simulink model "Smart_City_QCar1_self_driving_stack"  (R2024b)
settings: Solver=ode1  StartTime=0.0  StopTime=inf  FixedStep=Controller_Sample_Time  RelTol=1e-3  EnableMultiTasking=on
values from neighbouring files (symbols this model uses):
  angles_qcar1 = angles_new_qcar1(2: length (angles_new_qcar1), width (angles_new_qcar1)-5)    [Setup_QCar1and2_params.m]
  Audio_Sample_Time = 0.3    [Setup_QCar1and2_params.m]
  cal_pos = [0, 0, 0]    [Setup_QCar1and2_params.m]
  cameraStepSize = 3e-2    (= 0.03)    [Setup_QCar1and2_params.m]
  Cobra_Start = [0 0 0 0 0 0 0 0 0 0 0 0 ... (192000 elements, 192000x1)]    [QCar_Sounds.mat]
  Controller_Sample_Time = CSI_Sample_Time/10    (= 0.00166666666667)    [Setup_QCar1and2_params.m]
  CSI_Sample_Time = 1/60    (= 0.0166666666667)    [Setup_QCar1and2_params.m]
  GyroKF_P0 = eye(2)    [Setup_QCar1and2_params.m]
  GyroKF_Q = diag([0.01, 0.001])    [Setup_QCar1and2_params.m]
  GyroKF_R = 0.01    [Setup_QCar1and2_params.m]
  GyroKF_X0 = [0;0]    [Setup_QCar1and2_params.m]
  honk = [0.01708984375 0.0179443359375 0.018798828125 0.019775390625 0.0209655761719 0.0218505859375 0.0221557617188 0.0223693847656 0.022705078125 0.023681640625 0.0252075195312 0.0257263183594 ... (43568 elements, 21784x2)]    [QCar_Sounds.mat]
  ImageDisplay_Sample_Time = CSI_Sample_Time*6    (= 0.1)    [Setup_QCar1and2_params.m]
  Initialization_Time = 5    [Setup_QCar1and2_params.m]
  LiDAR_Sample_Time = CSI_Sample_Time*3    (= 0.05)    [Setup_QCar1and2_params.m]
  map_mask = [1 1 1 0 0 1 0]    [Setup_QCar1and2_params.m]
  NN_Sample_Time = RealSense_Sample_Time*1    (= 0.0333333333333)    [Setup_QCar1and2_params.m]
  path_x = [0.826 0.836 0.846 0.856 0.866 0.876 0.886 0.896 0.906 0.916 0.926 0.936 ... (740 elements, 740x1)]    [SDCS_Paths_7.mat]
  path_x2 = [-0.614 -0.604 -0.594 -0.584 -0.574 -0.564 -0.554 -0.544 -0.534 -0.524 -0.514 -0.504 ... (1090 elements, 1090x1)]    [SDCS_Paths_7.mat]
  path_x3 = [-0.614 -0.603821428571 -0.593642857143 -0.583464285714 -0.573285714286 -0.563107142857 -0.552928571429 -0.54275 -0.532571428571 -0.522392857143 -0.512214285714 -0.502035714286 ... (714 elements, 714x1)]    [SDCS_Paths_7.mat]
  path_x4 = [-0.614 -0.604 -0.594 -0.584 -0.574 -0.564 -0.554 -0.544 -0.534 -0.524 -0.514 -0.504 ... (1761 elements, 1761x1)]    [SDCS_Paths_7.mat]
  path_x5 = [1.436 1.42588571429 1.41577142857 1.40565714286 1.39554285714 1.38542857143 1.37531428571 1.3652 1.35508571429 1.34497142857 1.33485714286 1.32474285714 ... (574 elements, 574x1)]    [SDCS_Paths_7.mat]
  path_x6 = [1.436 1.42588571429 1.41577142857 1.40565714286 1.39554285714 1.38542857143 1.37531428571 1.3652 1.35508571429 1.34497142857 1.33485714286 1.32474285714 ... (1288 elements, 1288x1)]    [SDCS_Paths_7.mat]
  path_x7 = [-1.5778487585 -1.56959877056 -1.56127865467 -1.55288878259 -1.54442952915 -1.53590127231 -1.52730439309 -1.51863927561 -1.50990630701 -1.50110587746 -1.49223838016 -1.4833042113 ... (2260 elements, 2260x1)]    [SDCS_Paths_7.mat]
  path_y = [-1.0887 -1.0887 -1.0887 -1.0887 -1.0887 -1.0887 -1.0887 -1.0887 -1.0887 -1.0887 -1.0887 -1.0887 ... (740 elements, 740x1)]    [SDCS_Paths_7.mat]
  path_y2 = [-1.0887 -1.0887 -1.0887 -1.0887 -1.0887 -1.0887 -1.0887 -1.0887 -1.0887 -1.0887 -1.0887 -1.0887 ... (1090 elements, 1090x1)]    [SDCS_Paths_7.mat]
  path_y3 = [-1.0887 -1.0887 -1.0887 -1.0887 -1.0887 -1.0887 -1.0887 -1.0887 -1.0887 -1.0887 -1.0887 -1.0887 ... (714 elements, 714x1)]    [SDCS_Paths_7.mat]
  path_y4 = [-1.0887 -1.0887 -1.0887 -1.0887 -1.0887 -1.0887 -1.0887 -1.0887 -1.0887 -1.0887 -1.0887 -1.0887 ... (1761 elements, 1761x1)]    [SDCS_Paths_7.mat]
  path_y5 = [-0.8157 -0.8157 -0.8157 -0.8157 -0.8157 -0.8157 -0.8157 -0.8157 -0.8157 -0.8157 -0.8157 -0.8157 ... (574 elements, 574x1)]    [SDCS_Paths_7.mat]
  path_y6 = [-0.8157 -0.8157 -0.8157 -0.8157 -0.8157 -0.8157 -0.8157 -0.8157 -0.8157 -0.8157 -0.8157 -0.8157 ... (1288 elements, 1288x1)]    [SDCS_Paths_7.mat]
  path_y7 = [-0.614490295955 -0.61974988896 -0.624981792226 -0.630185771997 -0.635361595765 -0.640509032279 -0.645627851559 -0.6507178249 -0.655778724888 -0.660810325409 -0.665812401655 -0.670784730139 ... (2260 elements, 2260x1)]    [SDCS_Paths_7.mat]
  put_me_down = [0 0 0 0 0 0 0 0 0 0 0 0 ... (335870 elements, 167935x2)]    [QCar_Sounds.mat]
  qcar1_lidar_to_map_rotation = pi/2    (= 1.57079632679)    [Setup_QCar1and2_params.m]
  QCarEKF_L = 0.24    [Setup_QCar1and2_params.m]
  QCarEKF_P0 = eye(3)    [Setup_QCar1and2_params.m]
  QCarEKF_Q = diag([0.00001, 0.00001, 0.00001])    [Setup_QCar1and2_params.m]
  QCarEKF_R_combined = diag([0.1, 0.1, 0.01])    [Setup_QCar1and2_params.m]
  QCarEKF_R_heading = diag(0.1)    [Setup_QCar1and2_params.m]
  QcarKF_X0 = [0; 0; 0]    [Setup_QCar1and2_params.m]
  range_qcar1 = distance_new_qcar1(2: length (distance_new_qcar1), width (distance_new_qcar1)-5)    [Setup_QCar1and2_params.m]
  RealSense_Sample_Time = CSI_Sample_Time*2    (= 0.0333333333333)    [Setup_QCar1and2_params.m]
undefined symbols (not defined in the file or in its folder): DiscIntNeverNeededParam, gcbh, HIL, Joystick_Sample_Time, JPEG, Point, qc_get_step_size, video_display_show
libraries: quarc_library x63, simulink_extras x12, simulink x8
(part 2 of 5)

== system Smart_City_QCar1_self_driving_stack/QCar/QCar Control ==
  "Command (m/s, rad)" : Inport
  Model Heading (rad) : Inport  Port=2
  Hazard : Inport  Port=3
  Cos ^ : Inport  Port=4
  Car on : Inport  Port=5
  acceleration : Inport  Port=6
  Volume : Inport  Port=7
  Honk : Inport  Port=8
  Command : Saturate  UpperLimit=[3 .6]  LowerLimit=-[3 .6]
  Constant5 : Constant  Value=-inf
  Constant6 : Constant
  Data Type Conversion : DataTypeConversion  SaturateOnIntegerOverflow=off  RndMeth=Floor
  Demux : Demux  Outputs=2
  Demux1 : Demux  Outputs=2
  Display : Display
      settings: Decimation=100
  Display1 : Display
      settings: Decimation=100
  Memory : Memory
  Mux : Mux  Inputs=2
  Mux1 : Mux  Inputs=2
  Product : Product
  QCar I/O : Subsystem
  Rate Limiter Dynamic : simulink/Discontinuities/Rate Limiter Dynamic
  bicycleModel : Subsystem
  powerConsumptionMonitor : Subsystem
  speedController : Subsystem
  turnSpeedHandling : Subsystem
  Car Speed (m/s) : Outport
  "Pose_dot (m/s, m/s, rad/s)" : Outport  Port=2
  Battery (V) : Outport  Port=3
  Odometer (m) : Outport  Port=4
  Actual Steering : Outport  Port=5
  Current (A) : Outport  Port=6
  Commanded Speed : Outport  Port=7
  Gyro (rad/s) : Outport  Port=8
  wires:
  QCar I/O/2(batteryVoltage (V) [1]) -> Battery (V)/1, powerConsumptionMonitor/2(batteryVoltage (V) [1])
  powerConsumptionMonitor/1(motorPowerConsumption (W) [1]) -> Display/1
  QCar I/O/1(motorCurrent (A) [1]) -> Current (A)/1, powerConsumptionMonitor/1(motorCurrent (A) [1])
  Model Heading (rad)/1 -> bicycleModel/1(heading (rad))
  powerConsumptionMonitor/2(batteryLevel (%) [1]) -> Display1/1
  QCar I/O/4(gyroscopicRates (rad/s)) -> Gyro (rad/s)/1, bicycleModel/4(gyroscope (rad/s))
  bicycleModel/1("poseRate (m/s, m/s, rad/s)") -> "Pose_dot (m/s, m/s, rad/s)"/1
  Product/1 -> QCar I/O/1("motorCmd (%, rad) [2]"), bicycleModel/2("motorCommands (%, rad)"), Demux/1
  Car on/1 -> QCar I/O/2(Arm), speedController/1(arm (0,1)), Mux/1
  QCar I/O/5(Odometer) -> Odometer (m)/1
  [Speed] -> speedController/3(measuredSpeed (m/s))
  Demux/2 -> Actual Steering/1
  Hazard/1 -> Data Type Conversion/1
  Cos ^/1 -> turnSpeedHandling/2(Cos ^)
  Data Type Conversion/1 -> QCar I/O/3(Hazard)
  speedController/1(throttleCmd (%)) -> Product/2
  Mux/1 -> Product/1
  Constant6/1 -> Mux/2
  Volume/1 -> QCar I/O/4(Volume)
  QCar I/O/3(Speed (m/s)) -> [Speed], bicycleModel/3(carSpeed (m/s)), Car Speed (m/s)/1  "v"
  "Command (m/s, rad)"/1 -> Command/1
  Demux1/1 -> Rate Limiter Dynamic/2
  Rate Limiter Dynamic/1 -> Memory/1, Mux1/1
  Constant5/1 -> Rate Limiter Dynamic/3
  acceleration/1 -> Rate Limiter Dynamic/1
  Demux1/2 -> Mux1/2
  turnSpeedHandling/1(Commands) -> Demux1/1
  Mux1/1 -> speedController/2(desiredSpeed (m/s))
  Command/1 -> turnSpeedHandling/1(Commands in)
  Honk/1 -> QCar I/O/5(Honk)
  Memory/1 -> Commanded Speed/1

== system Smart_City_QCar1_self_driving_stack/QCar/QCar State Estimation ==
  v : Inport
  delta : Inport  Port=2
  x_gps : Inport  Port=3
  y_gps : Inport  Port=4
  th_gps : Inport  Port=5
  thd_gyro : Inport  Port=6
  newGPSData : Inport  Port=7
  Gyro Kalman Filter : MATLAB Function  TreatAsAtomicUnit=on
  QCar EKF : MATLAB Function  TreatAsAtomicUnit=on
  Xhat : Outport
  gyro_bias : Outport  Port=2
  wires:
  x_gps/1 -> QCar EKF/3(x_gps)
  y_gps/1 -> QCar EKF/4(y_gps)
  Gyro Kalman Filter/1(th_hat) -> QCar EKF/5(th_hat)
  newGPSData/1 -> QCar EKF/6(newGPSData), Gyro Kalman Filter/3(newGPSData)
  delta/1 -> QCar EKF/2(delta)
  thd_gyro/1 -> Gyro Kalman Filter/1(thd_gyro)
  v/1 -> QCar EKF/1(v)
  QCar EKF/1(Xhat) -> Xhat/1
  th_gps/1 -> Gyro Kalman Filter/2(th_gps)
  Gyro Kalman Filter/2(gyro_bias) -> gyro_bias/1

== system Smart_City_QCar1_self_driving_stack/QCar/Sensor Fusion - Complementary Filter ==
  note: One idead is to have the integrator reset if rate is high...
  note: stable gains Kp = 0.4*.4
  car speed : Inport
  rate : Inport  Port=2
  correction : Inport  Port=3
  Constant : Constant
  Constant1 : Constant  Value=5
  Constant2 : Constant  Value=.1
  Correction_Weight : Scope
  Display : Display
  Gain : Gain  Gain=[100 100 1]
  Integrator : Integrator  WrappedStateUpperValue=[20 20 pi]  WrappedStateLowerValue=-[20 20 pi]
  Integrator1 : Integrator  ExternalReset=level  LimitOutput=on  UpperSaturationLimit=.05*[1 1 1]*1  LowerSaturationLimit=-.05*[1 1 1]*1
  MATLAB Function : MATLAB Function  TreatAsAtomicUnit=on
  Manual Switch : ManualSwitch  CurrentSetting=0
  Product : Product
  Scope : Scope  NumInputPorts=2
  Subtract : Sum  Inputs=+-
  Subtract1 : Sum  Inputs=+-
  Subtract2 : Sum
  ki : Gain  Gain=[4 4 4]*1
  kp : Gain  Gain=[1 1 1]*.400*1
  estimate : Outport  VectorParamsAs1DForOutWhenUnconnected=off
  wires:
  Integrator/1 -> Subtract/1, estimate/1
  Subtract/1 -> ki/1, kp/1
  Integrator1/1 -> Scope/1, Subtract2/2
  kp/1 -> Scope/2, Subtract2/1
  Subtract1/1 -> Integrator/1
  ki/1 -> Integrator1/1
  correction/1 -> Subtract/2
  rate/1 -> Subtract1/1
  Manual Switch/1 -> Integrator1/2
  Constant/1 -> Manual Switch/1
  car speed/1 -> MATLAB Function/1(car_speed)
  MATLAB Function/1(correction_weight) -> Correction_Weight/1, Product/1, Display/1
  Subtract2/1 -> Gain/1
  Product/1 -> Subtract1/2
  Constant1/1 -> MATLAB Function/2(slope)
  Constant2/1 -> MATLAB Function/3(min_weight)
  Gain/1 -> Product/2

== system Smart_City_QCar1_self_driving_stack/QCar/Subsystem ==
  Angle : Inport
  Bias : Bias  Bias=pi  SaturateOnIntegerOverflow=off
  Bias1 : Bias  Bias=-pi  SaturateOnIntegerOverflow=off
  Constant1 : Constant  Value=2*pi
  Mod : Math  Operator=mod  SignedPower=on
  Mod_Angle : Outport
  wires:
  Mod/1 -> Bias1/1
  Constant1/1 -> Mod/2
  Bias/1 -> Mod/1
  Bias1/1 -> Mod_Angle/1
  Angle/1 -> Bias/1

== system Smart_City_QCar1_self_driving_stack/QCar/Subsystem1 ==
  Angle : Inport
  Bias : Bias  Bias=pi  SaturateOnIntegerOverflow=off
  Bias1 : Bias  Bias=-pi  SaturateOnIntegerOverflow=off
  Constant1 : Constant  Value=2*pi
  Mod : Math  Operator=mod  SignedPower=on
  Mod_Angle : Outport
  wires:
  Angle/1 -> Bias/1
  Bias1/1 -> Mod_Angle/1
  Bias/1 -> Mod/1
  Constant1/1 -> Mod/2
  Mod/1 -> Bias1/1

== system Smart_City_QCar1_self_driving_stack/Randomizer1/Subsystem1 ==
  Random Period : Inport
  Constant1 : Constant
  Less Than : RelationalOperator  Operator=<  OutDataTypeStr=boolean  RndMeth=Simplest  InputSameDT=off
  Mod : Math  Operator=mod
  Rate Transition : RateTransition  OutPortSampleTime=qc_get_step_size
  RisingEdge : Subsystem
  Time : quarc_library/Sources/Time/Time  time_source=Wall clock  sample_time=cameraStepSize*10
  RisingEdgeTrigger : Outport
  wires:
  Mod/1 -> Less Than/1
  Constant1/1 -> Less Than/2
  Rate Transition/1 -> Mod/1
  Less Than/1 -> RisingEdge/1(Input)
  Random Period/1 -> Mod/2
  Time/1 -> Rate Transition/1
  RisingEdge/1(RisingEdgeTrigger) -> RisingEdgeTrigger/1

== system Smart_City_QCar1_self_driving_stack/Randomizer1/select which which path set to use ==
  Trigger : TriggerPort  VariantControl=(inherit)
  Constant : Constant  Value=[1 1 0 1 0 0 1]
  Constant1 : Constant  Value=[0 0 1 0 1 1 0]
  Random Number : RandomNumber  Seed=7
  Switch : Switch  Criteria=u2 > Threshold  SaturateOnIntegerOverflow=off  InputSameDT=off
  map mask : Outport
  wires:
  Random Number/1 -> Switch/2
  Constant/1 -> Switch/1
  Constant1/1 -> Switch/3
  Switch/1 -> map mask/1

== system Smart_City_QCar1_self_driving_stack/Rate Timing Plots/monitorTiming ==
  note: Timing Performance
  note: moniorTiming Module:
      |
      | This subsystem outputs the sample time and computation time of the model.
      |
      | Outputs:
      | sampleTime (s) n/a : Sample time (unfiltered and filtered) in seconds.
      | computationTime (s) n/a : Computation time (unfiltered and filtered) in seconds.
      |
      | Usage:
      | Compare the Sample Time (s) output to a constant (qc_get_step_size) to monitor whether or not the desired sample time is being achieved. The Computation Time (s) values should be lower than the corresponding sample time value to ensure that the solver has enough time per time step.
  Computation Time : quarc_library/Sources/Time/Computation Time  sample_time=CSI_Sample_Time  use_model=on  use_cpu_time=off
  Constant : Constant  Value=CSI_Sample_Time  SampleTime=-1
  Mux : Mux  Inputs=3
  Sample Time : quarc_library/Sources/Time/Sample Time  Priority=-99  sample_time=CSI_Sample_Time
  Timing (s) : Outport  VectorParamsAs1DForOutWhenUnconnected=off
  wires:
  Computation Time/1 -> Mux/3
  Mux/1 -> Timing (s)/1
  Sample Time/1 -> Mux/1
  Constant/1 -> Mux/2

== system Smart_City_QCar1_self_driving_stack/Rate Timing Plots/monitorTiming1 ==
  note: moniorTiming Module:
      |
      | This subsystem outputs the sample time and computation time of the model.
      |
      | Outputs:
      | sampleTime (s) n/a : Sample time (unfiltered and filtered) in seconds.
      | computationTime (s) n/a : Computation time (unfiltered and filtered) in seconds.
      |
      | Usage:
      | Compare the Sample Time (s) output to a constant (qc_get_step_size) to monitor whether or not the desired sample time is being achieved. The Computation Time (s) values should be lower than the corresponding sample time value to ensure that the solver has enough time per time step.
  note: Timing Performance
  Computation Time : quarc_library/Sources/Time/Computation Time  sample_time=qc_get_step_size  use_model=on  use_cpu_time=off
  Constant : Constant  Value=qc_get_step_size  SampleTime=-1
  Mux : Mux  Inputs=3
  Sample Time : quarc_library/Sources/Time/Sample Time  Priority=-99  sample_time=qc_get_step_size
  Timing (s) : Outport  VectorParamsAs1DForOutWhenUnconnected=off
  wires:
  Constant/1 -> Mux/2
  Sample Time/1 -> Mux/1
  Mux/1 -> Timing (s)/1
  Computation Time/1 -> Mux/3

== system Smart_City_QCar1_self_driving_stack/Rate Timing Plots/monitorTiming2 ==
  note: moniorTiming Module:
      |
      | This subsystem outputs the sample time and computation time of the model.
      |
      | Outputs:
      | sampleTime (s) n/a : Sample time (unfiltered and filtered) in seconds.
      | computationTime (s) n/a : Computation time (unfiltered and filtered) in seconds.
      |
      | Usage:
      | Compare the Sample Time (s) output to a constant (qc_get_step_size) to monitor whether or not the desired sample time is being achieved. The Computation Time (s) values should be lower than the corresponding sample time value to ensure that the solver has enough time per time step.
  note: Timing Performance
  Computation Time : quarc_library/Sources/Time/Computation Time  sample_time=RealSense_Sample_Time  use_model=on  use_cpu_time=off
  Constant : Constant  Value=RealSense_Sample_Time  SampleTime=-1
  Mux : Mux  Inputs=3
  Sample Time : quarc_library/Sources/Time/Sample Time  Priority=-99  sample_time=RealSense_Sample_Time
  Timing (s) : Outport  VectorParamsAs1DForOutWhenUnconnected=off
  wires:
  Constant/1 -> Mux/2
  Sample Time/1 -> Mux/1
  Mux/1 -> Timing (s)/1
  Computation Time/1 -> Mux/3

== system Smart_City_QCar1_self_driving_stack/Rate Timing Plots/monitorTiming3 ==
  note: Timing Performance
  note: moniorTiming Module:
      |
      | This subsystem outputs the sample time and computation time of the model.
      |
      | Outputs:
      | sampleTime (s) n/a : Sample time (unfiltered and filtered) in seconds.
      | computationTime (s) n/a : Computation time (unfiltered and filtered) in seconds.
      |
      | Usage:
      | Compare the Sample Time (s) output to a constant (qc_get_step_size) to monitor whether or not the desired sample time is being achieved. The Computation Time (s) values should be lower than the corresponding sample time value to ensure that the solver has enough time per time step.
  Computation Time : quarc_library/Sources/Time/Computation Time  sample_time=ImageDisplay_Sample_Time  use_model=on  use_cpu_time=off
  Constant : Constant  Value=ImageDisplay_Sample_Time  SampleTime=-1
  Mux : Mux  Inputs=3
  Sample Time : quarc_library/Sources/Time/Sample Time  Priority=-99  sample_time=ImageDisplay_Sample_Time
  Timing (s) : Outport  VectorParamsAs1DForOutWhenUnconnected=off
  wires:
  Computation Time/1 -> Mux/3
  Mux/1 -> Timing (s)/1
  Sample Time/1 -> Mux/1
  Constant/1 -> Mux/2

== system Smart_City_QCar1_self_driving_stack/Rate Timing Plots/monitorTiming4 ==
  note: Timing Performance
  note: moniorTiming Module:
      |
      | This subsystem outputs the sample time and computation time of the model.
      |
      | Outputs:
      | sampleTime (s) n/a : Sample time (unfiltered and filtered) in seconds.
      | computationTime (s) n/a : Computation time (unfiltered and filtered) in seconds.
      |
      | Usage:
      | Compare the Sample Time (s) output to a constant (qc_get_step_size) to monitor whether or not the desired sample time is being achieved. The Computation Time (s) values should be lower than the corresponding sample time value to ensure that the solver has enough time per time step.
  Computation Time : quarc_library/Sources/Time/Computation Time  sample_time=Joystick_Sample_Time  use_model=on  use_cpu_time=off
  Constant : Constant  Value=Joystick_Sample_Time  SampleTime=-1
  Mux : Mux  Inputs=3
  Sample Time : quarc_library/Sources/Time/Sample Time  Priority=-99  sample_time=Joystick_Sample_Time
  Timing (s) : Outport  VectorParamsAs1DForOutWhenUnconnected=off
  wires:
  Computation Time/1 -> Mux/3
  Mux/1 -> Timing (s)/1
  Sample Time/1 -> Mux/1
  Constant/1 -> Mux/2

== system Smart_City_QCar1_self_driving_stack/Rate Timing Plots/monitorTiming5 ==
  note: moniorTiming Module:
      |
      | This subsystem outputs the sample time and computation time of the model.
      |
      | Outputs:
      | sampleTime (s) n/a : Sample time (unfiltered and filtered) in seconds.
      | computationTime (s) n/a : Computation time (unfiltered and filtered) in seconds.
      |
      | Usage:
      | Compare the Sample Time (s) output to a constant (qc_get_step_size) to monitor whether or not the desired sample time is being achieved. The Computation Time (s) values should be lower than the corresponding sample time value to ensure that the solver has enough time per time step.
  note: Timing Performance
  Computation Time : quarc_library/Sources/Time/Computation Time  sample_time=LiDAR_Sample_Time  use_model=on  use_cpu_time=off
  Constant : Constant  Value=LiDAR_Sample_Time  SampleTime=-1
  Mux : Mux  Inputs=3
  Sample Time : quarc_library/Sources/Time/Sample Time  Priority=-99  sample_time=LiDAR_Sample_Time
  Timing (s) : Outport  VectorParamsAs1DForOutWhenUnconnected=off
  wires:
  Constant/1 -> Mux/2
  Sample Time/1 -> Mux/1
  Mux/1 -> Timing (s)/1
  Computation Time/1 -> Mux/3

== system Smart_City_QCar1_self_driving_stack/Rate Timing Plots/monitorTiming6 ==
  note: Timing Performance
  note: moniorTiming Module:
      |
      | This subsystem outputs the sample time and computation time of the model.
      |
      | Outputs:
      | sampleTime (s) n/a : Sample time (unfiltered and filtered) in seconds.
      | computationTime (s) n/a : Computation time (unfiltered and filtered) in seconds.
      |
      | Usage:
      | Compare the Sample Time (s) output to a constant (qc_get_step_size) to monitor whether or not the desired sample time is being achieved. The Computation Time (s) values should be lower than the corresponding sample time value to ensure that the solver has enough time per time step.
  Computation Time : quarc_library/Sources/Time/Computation Time  sample_time=NN_Sample_Time  use_model=on  use_cpu_time=off
  Constant : Constant  Value=NN_Sample_Time  SampleTime=-1
  Mux : Mux  Inputs=3
  Sample Time : quarc_library/Sources/Time/Sample Time  Priority=-99  sample_time=NN_Sample_Time
  Timing (s) : Outport  VectorParamsAs1DForOutWhenUnconnected=off
  wires:
  Computation Time/1 -> Mux/3
  Mux/1 -> Timing (s)/1
  Sample Time/1 -> Mux/1
  Constant/1 -> Mux/2

== system Smart_City_QCar1_self_driving_stack/Rate Timing Plots/monitorTiming7 ==
  note: Timing Performance
  note: moniorTiming Module:
      |
      | This subsystem outputs the sample time and computation time of the model.
      |
      | Outputs:
      | sampleTime (s) n/a : Sample time (unfiltered and filtered) in seconds.
      | computationTime (s) n/a : Computation time (unfiltered and filtered) in seconds.
      |
      | Usage:
      | Compare the Sample Time (s) output to a constant (qc_get_step_size) to monitor whether or not the desired sample time is being achieved. The Computation Time (s) values should be lower than the corresponding sample time value to ensure that the solver has enough time per time step.
  Computation Time : quarc_library/Sources/Time/Computation Time  sample_time=1  use_model=on  use_cpu_time=off
  Constant : Constant  SampleTime=-1
  Mux : Mux  Inputs=3
  Sample Time : quarc_library/Sources/Time/Sample Time  Priority=-99  sample_time=1
  Timing (s) : Outport  VectorParamsAs1DForOutWhenUnconnected=off
  wires:
  Computation Time/1 -> Mux/3
  Mux/1 -> Timing (s)/1
  Sample Time/1 -> Mux/1
  Constant/1 -> Mux/2

== system Smart_City_QCar1_self_driving_stack/Rate Timing Plots/monitorTiming8 ==
  note: moniorTiming Module:
      |
      | This subsystem outputs the sample time and computation time of the model.
      |
      | Outputs:
      | sampleTime (s) n/a : Sample time (unfiltered and filtered) in seconds.
      | computationTime (s) n/a : Computation time (unfiltered and filtered) in seconds.
      |
      | Usage:
      | Compare the Sample Time (s) output to a constant (qc_get_step_size) to monitor whether or not the desired sample time is being achieved. The Computation Time (s) values should be lower than the corresponding sample time value to ensure that the solver has enough time per time step.
  note: Timing Performance
  Computation Time : quarc_library/Sources/Time/Computation Time  sample_time=Audio_Sample_Time  use_model=on  use_cpu_time=off
  Constant : Constant  Value=Audio_Sample_Time  SampleTime=-1
  Mux : Mux  Inputs=3
  Sample Time : quarc_library/Sources/Time/Sample Time  Priority=-99  sample_time=Audio_Sample_Time
  Timing (s) : Outport  VectorParamsAs1DForOutWhenUnconnected=off
  wires:
  Constant/1 -> Mux/2
  Sample Time/1 -> Mux/1
  Mux/1 -> Timing (s)/1
  Computation Time/1 -> Mux/3

== system Smart_City_QCar1_self_driving_stack/RealSense Camera/Newer Depth ==
  In1 : Inport
  Channel : quarc_library/Signal Routing/Channel  channel=0  buffer_size=1
  Image Compress : quarc_library/Image Processing/Generic/Image Compress  algorithm=JPEG  source=Internal dialog parameter  quality=quality  output_dim=-1
  Video Display : quarc_library/Multimedia/Video Display  Tag=Smart_City_QCar1_self_driving_stack/RealSense Camera/Newer Depth/Video Display  sample_time=sample_time  use_hardware=on
  wires:
  Image Compress/1 -> Channel/1
  In1/1 -> Image Compress/1
  Channel/1 -> Video Display/1

== system Smart_City_QCar1_self_driving_stack/RealSense Camera/RGB ==
  In1 : Inport
  Channel : quarc_library/Signal Routing/Channel  channel=1  buffer_size=1
  Image Compress : quarc_library/Image Processing/Generic/Image Compress  algorithm=JPEG  source=Internal dialog parameter  quality=quality  output_dim=-1
  Video Display : quarc_library/Multimedia/Video Display  Tag=Smart_City_QCar1_self_driving_stack/RealSense Camera/RGB/Video Display  sample_time=sample_time  use_hardware=on
  wires:
  Image Compress/1 -> Channel/1
  In1/1 -> Image Compress/1
  Channel/1 -> Video Display/1

== system Smart_City_QCar1_self_driving_stack/RealSense Camera/RealSense Capture ==
  AND : Logic  AllPortsSameDT=off  OutDataTypeStr=boolean
  AND1 : Logic  IconShape=distinctive  AllPortsSameDT=off  OutDataTypeStr=boolean
  Compare To Constant : simulink/Logic and Bit Operations/Compare To Constant  relop===  const=2  OutDataTypeStr=boolean
  Compare To Constant1 : simulink/Logic and Bit Operations/Compare To Constant  relop=>=  const=0  OutDataTypeStr=boolean
  Constant : Constant  Value=[1 0 0 0 0]
  Display : Display
  Display1 : Display
  Display2 : Display
  Image Compress : quarc_library/Image Processing/Generic/Image Compress  algorithm=JPEG  source=Internal dialog parameter  quality=50  output_dim=-1
  Memory : Memory  InheritSampleTime=on
  NN New : Scope
  NN Receive : Scope
  Rate Transition : RateTransition  OutPortSampleTime=NN_Sample_Time
  Stream Server : quarc_library/Communications/Basic/Stream Server  uri_source=Specify via dialog (do not evaluate)  uri=tcpip://remotehost:18999  send_buffer_size=640*360*3  receive_buffer_size=6*32  byte_order=little endian (Intel - LSB first)  optimization=Minimum latency  send_options=Send most recent data  receive_options=Receive most recent data  default_value=zeros(1,5,'single')  sample_time=NN_Sample_Time  active=off  implementation=Use blocking I/O in a separate thread  send_fifo_size=2  receive_fifo_size=2  send_priority=0  receive_priority=0  send_dimensions=on  receive_dimensions=off  max_dimensions=-1  data_type=single  type_expr=BusObject
      settings: AttributesFormatString="\"tcpip://remotehost:18999\""
  Switch : Switch  Criteria=u2 > Threshold  Threshold=0.5  SaturateOnIntegerOverflow=off  InputSameDT=off
  Terminator{,1..5} (6 alike) : Terminator
  Video3D Capture : quarc_library/Multimedia/Video3D Capture  object_name=RealSense  stream_type=Depth  stream_index=0  resolution=640 x 360  width=640  height=360  output_format=Distance in meters (HxW)  data_type=single  sample_time=RealSense_Sample_Time  camera_intrinsics=off  depth_scale=off  brightness_override=Do not override  brightness=50.0  contrast_override=Do not override  contrast=50.0  hue_override=Do not override  hue=50.0  saturation_override=Do not override  saturation=50.0  sharpness_override=Do not override  sharpness=50.0  gamma_override=Do not override  gamma=50.0  gain_override=Do not override  gain=50.0  backlightcompensation_override=Do not override  backlightcompensation=50.0  whitebalance_override=Automatic white balance  whitebalance=50.0  exposure_override=Automatic exposure  exposure=30.0  emitter=Enable laser emitter  preset=Do not set camera presets
  Video3D Capture1 : quarc_library/Multimedia/Video3D Capture  object_name=RealSense  stream_type=RGB  stream_index=0  resolution=640 x 360  width=640  height=360  output_format=MATLAB RGB (HxWx3)  data_type=uint8  sample_time=RealSense_Sample_Time*1  camera_intrinsics=off  depth_scale=off  brightness_override=Do not override  brightness=50.0  contrast_override=Do not override  contrast=50.0  hue_override=Do not override  hue=50.0  saturation_override=Do not override  saturation=50.0  sharpness_override=Do not override  sharpness=50.0  gamma_override=Do not override  gamma=50.0  gain_override=Do not override  gain=50.0  backlightcompensation_override=Do not override  backlightcompensation=50.0  whitebalance_override=Automatic white balance  whitebalance=50.0  exposure_override=Automatic exposure  exposure=30.0  emitter=Enable laser emitter  preset=Do not set camera presets
  Video3D Initialize : quarc_library/Multimedia/Video3D Initialize  object_name=RealSense  source=Device  identifier=0  file=sample.bag  sample_time=RealSense_Sample_Time  active=on
  New : Outport
  Depth : Outport  Port=2
  RGB Image : Outport  Port=3
  Sign Probabilities : Outport  Port=4
  wires:
  Video3D Capture/4 -> New/1
  Video3D Capture/2 -> Terminator4/1
  Video3D Capture/3 -> Terminator3/1
  Video3D Capture/1 -> Depth/1
  Video3D Initialize/1 -> Terminator/1
  Switch/1 -> Sign Probabilities/1
  Video3D Capture1/1 -> Rate Transition/1, RGB Image/1
  Constant/1 -> Switch/3
  Compare To Constant1/1 -> AND/2
  Stream Server/4 -> NN Receive/1, Switch/1
  Stream Server/2 -> Compare To Constant1/1, Display1/1
  Stream Server/5 -> NN New/1, Switch/2
  Stream Server/3 -> Terminator5/1
  Compare To Constant/1 -> AND/1
  Video3D Capture1/2 -> Terminator1/1
  Video3D Capture1/3 -> Terminator2/1
  Stream Server/1 -> Compare To Constant/1, Display/1
  Memory/1 -> AND1/2
  AND/1 -> Display2/1, Memory/1
  Video3D Capture1/4 -> AND1/1
  AND1/1 -> Stream Server/2
  Rate Transition/1 -> Image Compress/1
  Image Compress/1 -> Stream Server/1

== system Smart_City_QCar1_self_driving_stack/RealSense Camera/obstacleDetection Markham March 22 ==
  note: %
  note: m
  note: m
  note: %
  note: px
  note: px
  note: %
  note: %
  imageDepth : Inport
  steering (rad) : Inport  Port=2
  Enable : EnablePort  PropagateVarSize=During execution
  Add : Sum
  Bias : Constant  Value=0
  Box Color : Constant  Value=[255 0 0]
  Constant1 : Constant  Value=200
  Constant2 : Constant  Value=.15
  Constant3 : Constant
  Constant4 : Constant  Value=50
  Constant5 : Constant  Value=0.5
  Constant6 : Constant  Value=0.5
  Constant7 : Constant  Value=0.6
  Constant8 : Constant  Value=0.6
  Display : Display
  Draw Lines Module : MATLAB Function  TreatAsAtomicUnit=on
  Image Convert : quarc_library/Image Processing/Generic/Image Convert  input_format=MATLAB greyscale (HxW)  padding=0  output_format=MATLAB greyscale (HxW)  data_type=uint8
      settings: AttributesFormatString=(%<input_format>)  SourceProductName=QUARC Targets
  Saturation : Saturate  UpperLimit=2  LowerLimit=0.05
  Saturation1 : Saturate  UpperLimit=1  LowerLimit=0
  Scope : Scope
  Steering based image subselector : MATLAB Function  TreatAsAtomicUnit=on
  max white for 8m : Gain  Gain=1/2.5
  imageDepthForDisplay : Outport  VectorParamsAs1DForOutWhenUnconnected=off
  distance (m) : Outport  Port=2  VectorParamsAs1DForOutWhenUnconnected=off
  wires:
  Saturation1/1 -> Image Convert/1
  Constant6/1 -> Steering based image subselector/8(maxSteering)
  Steering based image subselector/2(distance) -> Add/1, Scope/1
  Constant5/1 -> Steering based image subselector/7(vertCenter)
  Constant4/1 -> Steering based image subselector/6(height)
  Constant1/1 -> Steering based image subselector/5(width)
  Constant3/1 -> Steering based image subselector/4(maxDistance)
  Constant2/1 -> Steering based image subselector/3(minDistance)
  steering (rad)/1 -> Steering based image subselector/2(steering)
  Draw Lines Module/1(img_out) -> imageDepthForDisplay/1
  Steering based image subselector/1(pts) -> Draw Lines Module/2(pts)
  Image Convert/1 -> Draw Lines Module/1(img_in)
  max white for 8m/1 -> Saturation1/1
  imageDepth/1 -> Steering based image subselector/1(depth), max white for 8m/1
  Bias/1 -> Add/2
  Add/1 -> Saturation/1, Display/1
  Saturation/1 -> distance (m)/1
  Box Color/1 -> Draw Lines Module/3(color)
  Constant7/1 -> Steering based image subselector/9(reduction)
  Constant8/1 -> Steering based image subselector/10(maxSteeringWidth)

== system Smart_City_QCar1_self_driving_stack/Speed & Steering Commander/Adaptive Cruise Control ==
  obstacleDistance (m) : Inport
  Desired Speed Command : Inport  Port=2
  Constant : Constant  Value=0.375
  Constant1 : Constant  Value=.4
  Constant2 : Constant  Value=0.6
  Less Than : RelationalOperator  Operator=<  OutDataTypeStr=boolean  RndMeth=Simplest  InputSameDT=off
  MATLAB Function : MATLAB Function  TreatAsAtomicUnit=on
  Scope : Scope  NumInputPorts=2
  Adjusted Speed Command : Outport  VectorParamsAs1DForOutWhenUnconnected=off
  Honk : Outport  Port=2
  wires:
  Constant2/1 -> MATLAB Function/3(nominal_tracking_distance)  "nominal tracking distance (m)"
  Constant/1 -> MATLAB Function/2(stop_distance)  "stop distance (m)"
  obstacleDistance (m)/1 -> Less Than/1, Scope/2, MATLAB Function/1(obstacle_distance)
  Constant1/1 -> Less Than/2
  Less Than/1 -> Honk/1
  MATLAB Function/1(speed_cmd) -> Scope/1, Adjusted Speed Command/1
  Desired Speed Command/1 -> MATLAB Function/4(nominal_speed)

== system Smart_City_QCar1_self_driving_stack/Speed & Steering Commander/Adaptive Cruise Control1 ==
  obstacleDistance (m) : Inport
  Desired Speed Command : Inport  Port=2
  Constant : Constant  Value=0.6
  Constant1 : Constant  Value=.4
  Constant2 : Constant
  Less Than : RelationalOperator  Operator=<  OutDataTypeStr=boolean  RndMeth=Simplest  InputSameDT=off
  MATLAB Function : MATLAB Function  TreatAsAtomicUnit=on
  Scope : Scope  NumInputPorts=2
  Adjusted Speed Command : Outport  VectorParamsAs1DForOutWhenUnconnected=off
  Honk : Outport  Port=2
  wires:
  Desired Speed Command/1 -> MATLAB Function/4(nominal_speed)
  MATLAB Function/1(speed_cmd) -> Adjusted Speed Command/1, Scope/1
  Less Than/1 -> Honk/1
  Constant1/1 -> Less Than/2
  obstacleDistance (m)/1 -> MATLAB Function/1(obstacle_distance), Scope/2, Less Than/1
  Constant/1 -> MATLAB Function/2(stop_distance)  "stop distance (m)"
  Constant2/1 -> MATLAB Function/3(nominal_tracking_distance)  "nominal tracking distance (m)"

== system Smart_City_QCar1_self_driving_stack/Speed & Steering Commander/Cross Track Controller ==
  closest point : Inport
  distance : Inport  Port=2
  xy : Inport  Port=3
  Heading : Inport  Port=4
  Commanded_Speed : Inport  Port=5
  Path : Inport  Port=6
  Constant : Constant  Value=0
  Constant1 : Constant
  Constant6 : Constant  Value=Initialization_Time
  Cos : Trigonometry  Operator=cos
  Cos1 : Trigonometry
  Cross Product : quarc_library/Math Operations/Vectors/Cross Product
      settings: SourceProductName=QUARC Targets
  Demux : Demux  Outputs=3
  Equal : RelationalOperator  Operator===  OutDataTypeStr=boolean  RndMeth=Simplest  InputSameDT=off
  Equal1 : RelationalOperator  Operator=~=  OutDataTypeStr=boolean  RndMeth=Simplest  InputSameDT=off
  Gain3 : Gain  Gain=.5
  Gain6 : Gain  Gain=2
  GreaterThan : RelationalOperator  Operator=<  OutDataTypeStr=boolean  RndMeth=Simplest  InputSameDT=off
  Integrator : Integrator  ExternalReset=level  LimitOutput=on  UpperSaturationLimit=.15  LowerSaturationLimit=-.15
  Integrator1 : Integrator  ExternalReset=level  LimitOutput=on  UpperSaturationLimit=1  LowerSaturationLimit=0
  Memory1 : Memory  InitialCondition=6  InheritSampleTime=on  LinearizeMemory=on  LinearizeAsDelay=on
  Mux : Mux  Inputs=3
  Mux1 : Mux  Inputs=2
  Mux2 : Mux  Inputs=2
  OR : Logic  Operator=OR  Inputs=3  IconShape=distinctive  AllPortsSameDT=off  OutDataTypeStr=boolean
  Product : Product
  Product3 : Product
  Radians to Degrees : simulink_extras/Transformations/Radians to Degrees
  Saturation1 : Saturate  UpperLimit=.15  LowerLimit=-.15
  Scope1 : Scope  NumInputPorts=2
  Sign : Signum
  Sum : Sum  Inputs=+-
  Sum2 : Sum
  Time1 : quarc_library/Sources/Time/Time  time_source=Wall clock  sample_time=qc_get_step_size
  steering correction : Outport
  wires:
  Heading/1 -> Cos1/1, Cos/1
  Cos/1 -> Mux/1
  Cos1/1 -> Mux/2
  xy/1 -> Sum/2
  closest point/1 -> Sum/1
  Sum/1 -> Mux1/1
  Mux1/1 -> Cross Product/2
  Mux/1 -> Cross Product/1
  Cross Product/1 -> Demux/1
  Demux/3 -> Sign/1
  Sign/1 -> Product3/1
  Gain6/1 -> Integrator/1
  Product3/1 -> Gain3/1, Gain6/1
  Integrator/1 -> Mux2/1, Sum2/1
  Saturation1/1 -> Mux2/2, Sum2/2
  distance/1 -> Product3/2
  Sum2/1 -> steering correction/1
  Commanded_Speed/1 -> Equal/1
  Constant/1 -> Equal/2
  Path/1 -> Equal1/2, Memory1/1
  Memory1/1 -> Equal1/1
  Equal1/1 -> OR/2
  Equal/1 -> OR/1
  OR/1 -> Scope1/1, Integrator1/2, Integrator/2
  Constant1/1 -> Integrator1/1
  Product/1 -> Saturation1/1
  Gain3/1 -> Product/1
  Integrator1/1 -> Product/2
  Mux2/1 -> Radians to Degrees/1
  Radians to Degrees/1 -> Scope1/2
  Time1/1 -> GreaterThan/1
  Constant6/1 -> GreaterThan/2
  GreaterThan/1 -> OR/3

== system Smart_City_QCar1_self_driving_stack/Speed & Steering Commander/LiDAR Steering ==
  xy_command : Inport
  xy : Inport  Port=2
  heading : Inport  Port=3
  Direction Vector Generator : Subsystem
  Display1 : Display
      settings: Decimation=100
  Gain1 : Gain
  Radians to Degrees1 : simulink_extras/Transformations/Radians to Degrees
  Steering Commander : MATLAB Function  TreatAsAtomicUnit=on
  distance : Outport
  LiDAR Steering : Outport  Port=2
  wires:
  Direction Vector Generator/1(distance) -> distance/1
  xy_command/1 -> Direction Vector Generator/1(xy_command)
  Direction Vector Generator/2(aoa) -> Radians to Degrees1/1, Steering Commander/1(aoa)
  Gain1/1 -> LiDAR Steering/1
  Radians to Degrees1/1 -> Display1/1
  xy/1 -> Direction Vector Generator/2(xy)
  heading/1 -> Direction Vector Generator/3(heading)
  Steering Commander/1(steering) -> Gain1/1

== system Smart_City_QCar1_self_driving_stack/Speed & Steering Commander/Path Commander ==
  path : Inport
  xy : Inport  Port=2
  look_ahead_d : Inport  Port=3
  Allowable Paths Mask : Gain  Gain=map_mask
  Allowable distance from path for viable paths : Constant  Value=0.05
  Data Type Conversion : DataTypeConversion  SaturateOnIntegerOverflow=off  RndMeth=Floor
  Display : Display
  "Distance  " : Scope
  Duration (s) within allowable distance before viable path detected : Constant  Value=0.2
  Less Than Threshold : Subsystem
  Multiport Switch : MultiPortSwitch  Inputs=7  DiagnosticForDefault=None  SaturateOnIntegerOverflow=off  InputSameDT=off
  Multiport Switch1 : MultiPortSwitch  Inputs=7  DiagnosticForDefault=None  SaturateOnIntegerOverflow=off  InputSameDT=off
  Multiport Switch2 : MultiPortSwitch  Inputs=7  DiagnosticForDefault=None  SaturateOnIntegerOverflow=off  InputSameDT=off
  Mux : Mux  Inputs=7
  Path 1  Look Ahead Generator : Subsystem
  Path 2  Look Ahead Generator : Subsystem
  Path 3  Look Ahead Generator : Subsystem
  Path 4  Look Ahead Generator : Subsystem
  Path 5  Look Ahead Generator : Subsystem
  Path 6  Look Ahead Generator : Subsystem
  Path 7  Look Ahead Generator : Subsystem
  Terminator : Terminator
  xy_cmd : Outport
  Path_Options : Outport  Port=2
  closest point : Outport  Port=3
  distance : Outport  Port=4
  wires:
  look_ahead_d/1 -> Path 7  Look Ahead Generator/2(look_ahead_d), Path 6  Look Ahead Generator/2(look_ahead_d), Path 5  Look Ahead Generator/2(look_ahead_d), Path 4  Look Ahead Generator/2(look_ahead_d), Path 3  Look Ahead Generator/2(look_ahead_d), Path 2  Look Ahead Generator/2(look_ahead_d), Path 1  Look Ahead Generator/2(look_ahead_d)
  path/1 -> Multiport Switch2/1, Multiport Switch1/1, Multiport Switch/1
  Path 1  Look Ahead Generator/1(xy_cmd) -> Multiport Switch/2
  Path 2  Look Ahead Generator/1(xy_cmd) -> Multiport Switch/3
  Multiport Switch/1 -> xy_cmd/1
  Path 3  Look Ahead Generator/1(xy_cmd) -> Multiport Switch/4
  Path 4  Look Ahead Generator/1(xy_cmd) -> Multiport Switch/5
  Path 1  Look Ahead Generator/3(distance) -> Multiport Switch2/2, Mux/1
  Path 2  Look Ahead Generator/3(distance) -> Multiport Switch2/3, Mux/2
  Path 3  Look Ahead Generator/3(distance) -> Multiport Switch2/4, Mux/3
  Path 4  Look Ahead Generator/3(distance) -> Multiport Switch2/5, Mux/4
  Mux/1 -> Less Than Threshold/1(Distances), "Distance  "/1
  Allowable distance from path for viable paths/1 -> Less Than Threshold/2(Distance Threshold)
  Duration (s) within allowable distance before viable path detected/1 -> Less Than Threshold/3(Duration Threshold)
  Less Than Threshold/1(elapsed) -> Data Type Conversion/1, Display/1
  Allowable Paths Mask/1 -> Path_Options/1
  Data Type Conversion/1 -> Allowable Paths Mask/1
  Path 5  Look Ahead Generator/1(xy_cmd) -> Multiport Switch/6
  Path 6  Look Ahead Generator/1(xy_cmd) -> Multiport Switch/7
  Path 5  Look Ahead Generator/3(distance) -> Multiport Switch2/6, Mux/5
  Path 6  Look Ahead Generator/3(distance) -> Multiport Switch2/7, Mux/6
  Path 1  Look Ahead Generator/2(closest_point) -> Multiport Switch1/2
  Path 2  Look Ahead Generator/2(closest_point) -> Multiport Switch1/3
  Path 3  Look Ahead Generator/2(closest_point) -> Multiport Switch1/4
  Path 4  Look Ahead Generator/2(closest_point) -> Multiport Switch1/5
  Path 5  Look Ahead Generator/2(closest_point) -> Multiport Switch1/6
  Path 6  Look Ahead Generator/2(closest_point) -> Multiport Switch1/7
  Multiport Switch1/1 -> closest point/1
  Multiport Switch2/1 -> distance/1
  xy/1 -> Path 7  Look Ahead Generator/1(xy), Path 6  Look Ahead Generator/1(xy), Path 5  Look Ahead Generator/1(xy), Path 4  Look Ahead Generator/1(xy), Path 3  Look Ahead Generator/1(xy), Path 2  Look Ahead Generator/1(xy), Path 1  Look Ahead Generator/1(xy)
  Path 7  Look Ahead Generator/1(xy_cmd) -> Multiport Switch/8
  Path 7  Look Ahead Generator/2(closest_point) -> Multiport Switch1/8
  Path 7  Look Ahead Generator/3(distance) -> Mux/7, Multiport Switch2/8
  Less Than Threshold/2(time) -> Terminator/1

== system Smart_City_QCar1_self_driving_stack/Speed & Steering Commander/Sign Finder ==
  Signs : Inport
  Constant1 : Constant  Value=.8
  Constant15 : Constant  Value=.9
  Constant16 : Constant  Value=.06
  Constant2 : Constant  Value=.06
  Demux : Demux  Outputs=5
  Greater Than Threshold : Subsystem
  Greater Than Threshold1 : Subsystem
  Stop Sign : Outport
  Slow Sign : Outport  Port=2
  wires:
  Signs/1 -> Demux/1
  Constant16/1 -> Greater Than Threshold/3(Duration)
  Constant15/1 -> Greater Than Threshold/2(Threshold)
  Demux/4 -> Greater Than Threshold/1(Signal)
  Greater Than Threshold/1(elapsed) -> Stop Sign/1
  Greater Than Threshold1/1(elapsed) -> Slow Sign/1
  Demux/3 -> Greater Than Threshold1/1(Signal)
  Constant1/1 -> Greater Than Threshold1/2(Threshold)
  Constant2/1 -> Greater Than Threshold1/3(Duration)

== system Smart_City_QCar1_self_driving_stack/Speed & Steering Commander/Traffic Zone 1 ==
  note: select the control variable
  xy : Inport
  speed in : Inport  Port=2
  Traffic Light : Inport  Port=3
  1 is green : Display
  AND : Logic  Inputs=4  IconShape=distinctive  AllPortsSameDT=off  OutDataTypeStr=boolean
  Bias : Bias  Bias=-0.4  SaturateOnIntegerOverflow=off
  Constant13 : Constant  Value=[-0.61 -1.21]
  Constant14 : Constant  Value=[-0.4 -0.86]
  Constant3 : Constant  Value=.1
  Demux : Demux  Outputs=2
  Demux1 : Demux  Outputs=2
  Demux2 : Demux  Outputs=2
  Gain : Gain
  Greater Than Threshold : Subsystem
  Less Than Threshold : Subsystem
  MATLAB Function2 : MATLAB Function  TreatAsAtomicUnit=on
  Memory7 : Memory  InitialCondition=1  InheritSampleTime=on  LinearizeMemory=on  LinearizeAsDelay=on
  Saturation : Saturate  UpperLimit=1  LowerLimit=0
  "Speed " : Scope
  Speed Multi : Scope
  Traffic State : Display
  in zone : Display
  Speed Out : Outport
  wires:
  xy/1 -> Demux2/1, Less Than Threshold/1(Signal), Greater Than Threshold/1(Signal)
  Constant3/1 -> Less Than Threshold/3(Duration), Greater Than Threshold/3(Duration)
  Constant13/1 -> Greater Than Threshold/2(Threshold)
  Constant14/1 -> Less Than Threshold/2(Threshold)
  Greater Than Threshold/1(elapsed) -> Demux/1
  Demux/2 -> AND/2
  Demux/1 -> AND/1
  Less Than Threshold/1(elapsed) -> Demux1/1
  Demux1/2 -> AND/4
  Demux1/1 -> AND/3
  Demux2/1 -> Bias/1
  Bias/1 -> Gain/1
  Gain/1 -> Saturation/1
  MATLAB Function2/1(Traffic_State) -> Memory7/1, Traffic State/1
  Memory7/1 -> MATLAB Function2/1(Previous_State)
  speed in/1 -> MATLAB Function2/2(Speed_In)
  AND/1 -> MATLAB Function2/4(In_Zone), in zone/1
  Saturation/1 -> Speed Multi/1, MATLAB Function2/3(Speed_Multi)
  MATLAB Function2/2(Speed_Out) -> Speed Out/1, "Speed "/1
  Traffic Light/1 -> 1 is green/1, MATLAB Function2/5(Traffic_Light)

== system Smart_City_QCar1_self_driving_stack/Speed & Steering Commander/Traffic Zone 2 ==
  note: select the control variable
  xy : Inport
  speed in : Inport  Port=2
  Traffic Light : Inport  Port=3
  1 is green : Display
  AND : Logic  Inputs=4  IconShape=distinctive  AllPortsSameDT=off  OutDataTypeStr=boolean
  Bias : Bias  Bias=0.8  SaturateOnIntegerOverflow=off
  Constant13 : Constant  Value=[0.75 -0.9]
  Constant14 : Constant  Value=[1.35 -0.65]
  Constant3 : Constant  Value=.1
  Demux : Demux  Outputs=2
  Demux1 : Demux  Outputs=2
  Demux2 : Demux  Outputs=2
  Gain : Gain  Gain=-1
  Greater Than Threshold : Subsystem
  Less Than Threshold : Subsystem
  MATLAB Function2 : MATLAB Function  TreatAsAtomicUnit=on
  Memory7 : Memory  InitialCondition=1  InheritSampleTime=on  LinearizeMemory=on  LinearizeAsDelay=on
  Saturation : Saturate  UpperLimit=1  LowerLimit=0
  "Speed " : Scope
  Speed Multi : Scope
  Traffic State : Display
  in zone : Display
  Speed Out : Outport
  wires:
  MATLAB Function2/2(Speed_Out) -> "Speed "/1, Speed Out/1
  Saturation/1 -> MATLAB Function2/3(Speed_Multi), Speed Multi/1
  AND/1 -> in zone/1, MATLAB Function2/4(In_Zone)
  speed in/1 -> MATLAB Function2/2(Speed_In)
  Memory7/1 -> MATLAB Function2/1(Previous_State)
  MATLAB Function2/1(Traffic_State) -> Traffic State/1, Memory7/1
  Gain/1 -> Saturation/1
  Bias/1 -> Gain/1
  Demux2/1 -> Bias/1
  Demux1/1 -> AND/3
  Demux1/2 -> AND/4
  Less Than Threshold/1(elapsed) -> Demux1/1
  Demux/1 -> AND/1
  Demux/2 -> AND/2
  Greater Than Threshold/1(elapsed) -> Demux/1
  Constant14/1 -> Less Than Threshold/2(Threshold)
  Constant13/1 -> Greater Than Threshold/2(Threshold)
  Constant3/1 -> Greater Than Threshold/3(Duration), Less Than Threshold/3(Duration)
  xy/1 -> Greater Than Threshold/1(Signal), Less Than Threshold/1(Signal), Demux2/1
  Traffic Light/1 -> 1 is green/1, MATLAB Function2/5(Traffic_Light)

== system Smart_City_QCar1_self_driving_stack/Speed & Steering Commander/xy signal maker ==
  xy 1 : Inport
  xy 2 : Inport  Port=2
  Demux1 : Demux  Outputs=2
  Demux2 : Demux  Outputs=2
  Mux : Mux  Inputs=2
  Mux1 : Mux  Inputs=2
  Rate Transition1 : RateTransition  OutPortSampleTime=ImageDisplay_Sample_Time
  Rate Transition2 : RateTransition  OutPortSampleTime=ImageDisplay_Sample_Time
  x : Outport
  y : Outport  Port=2
  wires:
  Demux2/1 -> Mux/2
  Demux1/2 -> Mux1/1
  Demux1/1 -> Mux/1
  Demux2/2 -> Mux1/2
  Mux/1 -> x/1
  Mux1/1 -> y/1
  xy 1/1 -> Rate Transition1/1
  Rate Transition1/1 -> Demux1/1
  xy 2/1 -> Rate Transition2/1
  Rate Transition2/1 -> Demux2/1

== system Smart_City_QCar1_self_driving_stack/QCar/Fusion Comparison & Kalman Estimator/Angle mod1 ==
  Angle : Inport
  Bias : Bias  Bias=180  SaturateOnIntegerOverflow=off
  Bias1 : Bias  Bias=-180  SaturateOnIntegerOverflow=off
  Constant1 : Constant  Value=360
  Mod : Math  Operator=mod  SignedPower=on
  Mod_Angle : Outport
  wires:
  Angle/1 -> Bias/1
  Bias1/1 -> Mod_Angle/1
  Bias/1 -> Mod/1
  Constant1/1 -> Mod/2
  Mod/1 -> Bias1/1

== system Smart_City_QCar1_self_driving_stack/QCar/LiDAR/Match Scans ==
  Current_Distance : Inport
  Angles : Inport  Port=2
  Ref_Distance : Inport  Port=3
  Ref_Angles : Inport  Port=4
  absolute_scan : Inport  Port=5
  Previous Estimate : Inport  Port=6
  Enable : EnablePort  PropagateVarSize=During execution
  Constant : Constant  Value=[6 6 2*pi]
  Constant1 : Constant  Value=[1 1 pi/2]
  Data Type Conversion : DataTypeConversion  SaturateOnIntegerOverflow=off  RndMeth=Floor
  Data Type Conversion1 : DataTypeConversion  SaturateOnIntegerOverflow=off  RndMeth=Floor
  Demux : Demux  Outputs=2
  Display : Display
  Gain : Gain  Gain=[1 -1 -1]
  Gain1 : Gain  Gain=[1 -1 -1]
  LIDAR Scan Match : quarc_library/Image Processing/Generic/LIDAR Scan Match  mode=Variable-size input  resolution=35  max_range=6  use_initial_pose=on
      settings: SourceProductName=QUARC Targets
  MATLAB Function : MATLAB Function  TreatAsAtomicUnit=on
  Memory : Memory  InitialCondition=[0 0 0]  InheritSampleTime=on  LinearizeMemory=on  LinearizeAsDelay=on
  Pose Deltas : Scope
  Scope : Scope
  Subtract : Sum  Inputs=+-
  Switch : Switch  Criteria=u2 > Threshold  Threshold=.5  SaturateOnIntegerOverflow=off  InputSameDT=off
  Width : Width
  pose : Outport
  score : Outport  Port=2
  wires:
  LIDAR Scan Match/1 -> Memory/1, Subtract/1, Gain/1  "pose"
  Ref_Distance/1 -> LIDAR Scan Match/3
  Ref_Angles/1 -> LIDAR Scan Match/4
  Gain/1 -> Data Type Conversion/1
  LIDAR Scan Match/2 -> score/1
  Memory/1 -> Subtract/2
  absolute_scan/1 -> Switch/2
  Switch/1 -> Demux/1, Display/1
  Demux/1 -> LIDAR Scan Match/6
  Demux/2 -> LIDAR Scan Match/7
  Constant/1 -> Switch/1
  Constant1/1 -> Switch/3
  Data Type Conversion/1 -> pose/1
  Angles/1 -> MATLAB Function/2(angles)
  Current_Distance/1 -> MATLAB Function/1(range)
  MATLAB Function/1(new_range) -> Width/1, LIDAR Scan Match/1
  MATLAB Function/2(new_angles) -> LIDAR Scan Match/2
  Width/1 -> Scope/1
  Subtract/1 -> Pose Deltas/1
  Previous Estimate/1 -> Data Type Conversion1/1
  Gain1/1 -> LIDAR Scan Match/5
  Data Type Conversion1/1 -> Gain1/1

== system Smart_City_QCar1_self_driving_stack/QCar/LiDAR/RisingEdge ==
  Input : Inport
  Logical Operator1 : Logic  AllPortsSameDT=off
  Logical Operator2 : Logic  Operator=NOT  AllPortsSameDT=off
  Memory : Memory  InheritSampleTime=on  LinearizeMemory=on
  RisingEdgeTrigger : Outport  VectorParamsAs1DForOutWhenUnconnected=off
  wires:
  Logical Operator1/1 -> RisingEdgeTrigger/1
  Logical Operator2/1 -> Logical Operator1/2
  Memory/1 -> Logical Operator2/1
  Input/1 -> Logical Operator1/1, Memory/1
